simulink subsystem "CL1MGR"  (R2024b)
settings: Solver=VariableStepAuto  StartTime=0.0  StopTime=10.0  RelTol=1e-3
settings Model: Creator=jeonghyun  LastModifiedBy=jeonghyun

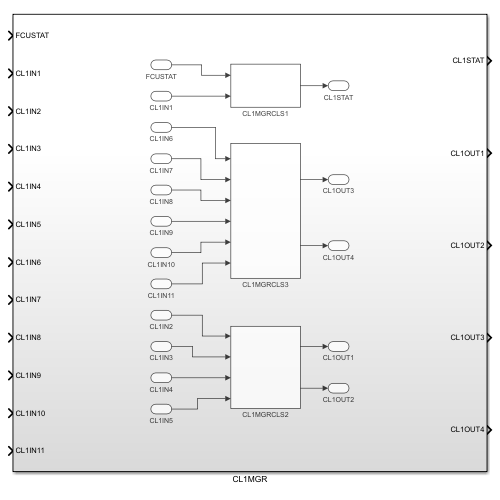
[thumbnail: Simulink's stored preview of the top-level diagram]
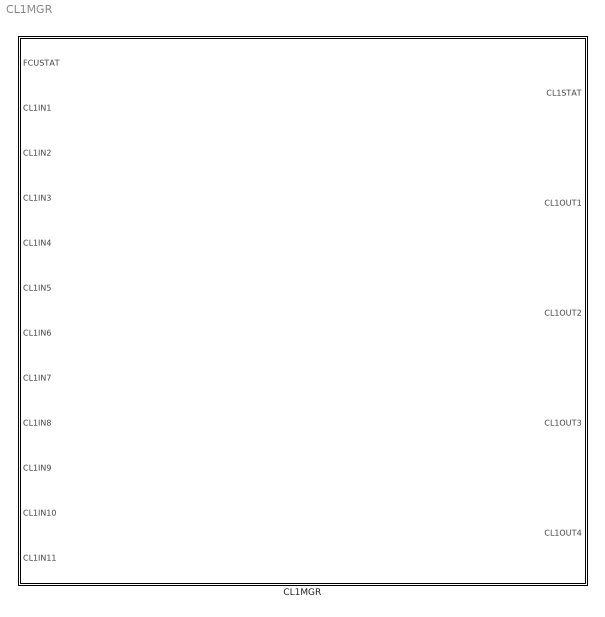
== system CL1MGR ==
  CL1MGR : Subsystem

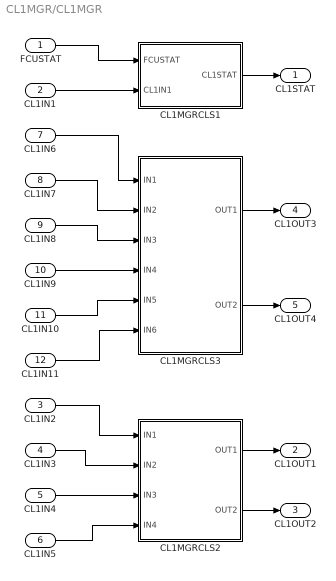
== system CL1MGR/CL1MGR ==
  FCUSTAT : Inport
  CL1IN1 : Inport  Port=2
  CL1IN2 : Inport  Port=3
  CL1IN3 : Inport  Port=4
  CL1IN4 : Inport  Port=5
  CL1IN5 : Inport  Port=6
  CL1IN6 : Inport  Port=7
  CL1IN7 : Inport  Port=8
  CL1IN8 : Inport  Port=9
  CL1IN9 : Inport  Port=10
  CL1IN10 : Inport  Port=11
  CL1IN11 : Inport  Port=12
  CL1MGRCLS1 : Subsystem
  CL1MGRCLS2 : Subsystem
  CL1MGRCLS3 : Subsystem
  CL1STAT : Outport
  CL1OUT1 : Outport  Port=2
  CL1OUT2 : Outport  Port=3
  CL1OUT3 : Outport  Port=4
  CL1OUT4 : Outport  Port=5
  wires:
  FCUSTAT/1 -> CL1MGRCLS1/1(FCUSTAT)
  CL1IN4/1 -> CL1MGRCLS2/3(IN3)
  CL1IN1/1 -> CL1MGRCLS1/2(CL1IN1)
  CL1MGRCLS3/1(OUT1) -> CL1OUT3/1
  CL1IN5/1 -> CL1MGRCLS2/4(IN4)
  CL1IN7/1 -> CL1MGRCLS3/2(IN2)
  CL1IN6/1 -> CL1MGRCLS3/1(IN1)
  CL1IN9/1 -> CL1MGRCLS3/4(IN4)
  CL1IN8/1 -> CL1MGRCLS3/3(IN3)
  CL1IN11/1 -> CL1MGRCLS3/6(IN6)
  CL1IN10/1 -> CL1MGRCLS3/5(IN5)
  CL1IN2/1 -> CL1MGRCLS2/1(IN1)
  CL1IN3/1 -> CL1MGRCLS2/2(IN2)
  CL1MGRCLS1/1(CL1STAT) -> CL1STAT/1
  CL1MGRCLS3/2(OUT2) -> CL1OUT4/1
  CL1MGRCLS2/1(OUT1) -> CL1OUT1/1
  CL1MGRCLS2/2(OUT2) -> CL1OUT2/1

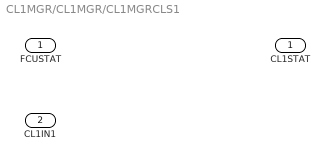
== system CL1MGR/CL1MGR/CL1MGRCLS1 ==
  FCUSTAT : Inport
  CL1IN1 : Inport  Port=2
  CL1STAT : Outport

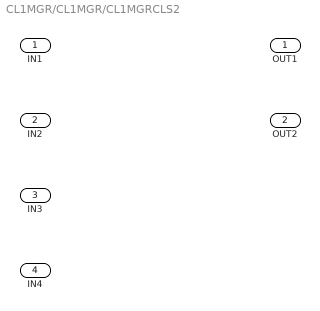
== system CL1MGR/CL1MGR/CL1MGRCLS2 ==
  IN1 : Inport
  IN2 : Inport  Port=2
  IN3 : Inport  Port=3
  IN4 : Inport  Port=4
  OUT1 : Outport
  OUT2 : Outport  Port=2

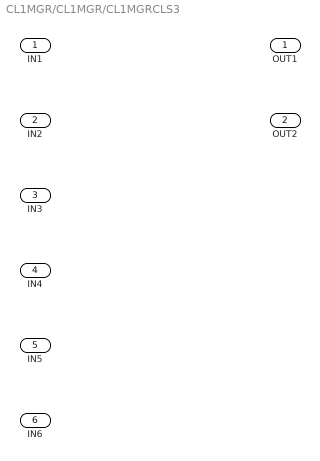
== system CL1MGR/CL1MGR/CL1MGRCLS3 ==
  IN1 : Inport
  IN2 : Inport  Port=2
  IN3 : Inport  Port=3
  IN4 : Inport  Port=4
  IN5 : Inport  Port=5
  IN6 : Inport  Port=6
  OUT1 : Outport
  OUT2 : Outport  Port=2
